simulink model "galipeur"  (R2017a)
settings: Solver=FixedStepAuto  StartTime=0.0  StopTime=inf  FixedStep=0.01  MaxStep=0.05  RelTol=1e-3
model workspace (MAT data in the model file):
  Jz = 3
  alpha0 = 1.57079632679
  alpha1 = 3.66519142919
  alpha2 = 5.75958653158
  mass = 3
  radius = 0.3
undefined symbols (not defined in the file): DiscIntNeverNeededParam
libraries: galipeur_lib x6, simulink x1
settings Model: Creator=jdam  LastModifiedBy=jdam
settings SolverCC: InitialStep=0.05

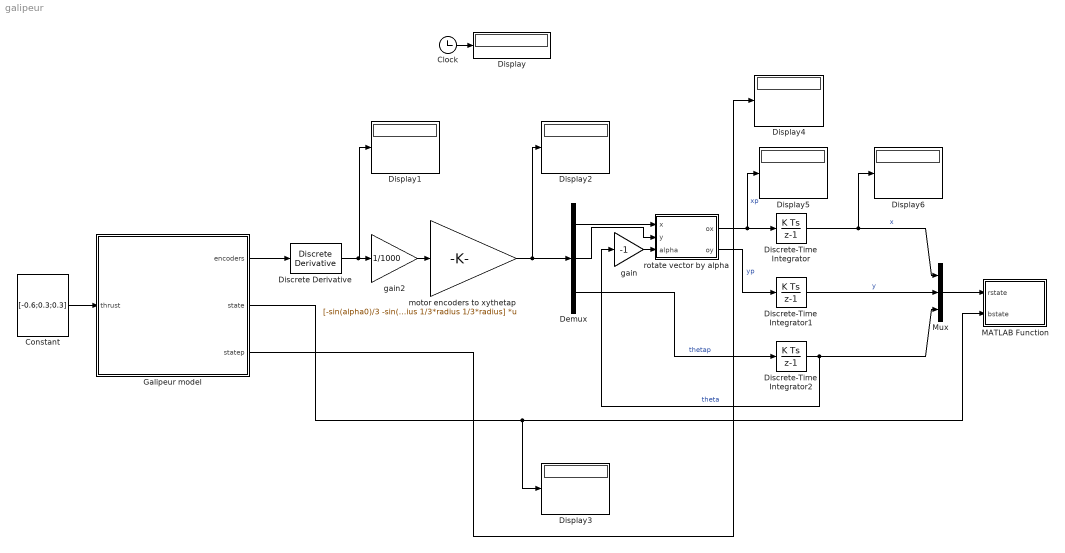
== system galipeur ==
  Clock : Clock
  Constant : Constant  Value=[-0.6;0.3;0.3]  VectorParams1D=off
  Demux : Demux  Outputs=3
  Discrete Derivative : simulink/Discrete/Discrete Derivative  gainval=1.0  ICPrevScaledInput=0.0  OutMin=[]  OutMax=[]  OutDataType=fixdt(1, 16)  OutScaling=2^-10  DoSatur=off
  Discrete-Time Integrator : DiscreteIntegrator  InitialConditionSetting=State (most efficient)  SampleTime=-1  ICPrevOutput=DiscIntNeverNeededParam  ICPrevScaledInput=DiscIntNeverNeededParam
  Discrete-Time Integrator1 : DiscreteIntegrator  InitialConditionSetting=State (most efficient)  SampleTime=-1  ICPrevOutput=DiscIntNeverNeededParam  ICPrevScaledInput=DiscIntNeverNeededParam
  Discrete-Time Integrator2 : DiscreteIntegrator  InitialConditionSetting=State (most efficient)  SampleTime=-1  ICPrevOutput=DiscIntNeverNeededParam  ICPrevScaledInput=DiscIntNeverNeededParam
  Display{,1..6} (7 alike) : Display
  Galipeur model : Subsystem
  MATLAB Function : MATLAB Function  TreatAsAtomicUnit=on
  Mux : Mux  Inputs=3
  gain : Gain  Gain=-1
  gain2 : Gain  Gain=1/1000
  motor encoders to xythetap : Gain  Gain=[-sin(alpha0)/3 -sin(alpha1)/3 -sin(alpha2)/3; cos(alpha0)/3 cos(alpha1)/3 cos(alpha2)/3; 1/3*radius 1/3*radius 1/3*radius]  Multiplication=Matrix(K*u) (u vector)
  rotate vector by alpha : MATLAB Function  TreatAsAtomicUnit=on
  wires:
  Clock/1 -> Display/1
  Constant/1 -> Galipeur model/1(thrust)
  Galipeur model/1(encoders) -> Discrete Derivative/1
  Discrete Derivative/1 -> Display1/1, gain2/1
  Demux/1 -> rotate vector by alpha/1(x)
  Demux/2 -> rotate vector by alpha/2(y)
  rotate vector by alpha/1(ox) -> Display5/1, Discrete-Time Integrator/1  "xp"
  rotate vector by alpha/2(oy) -> Discrete-Time Integrator1/1  "yp"
  gain/1 -> rotate vector by alpha/3(alpha)
  Discrete-Time Integrator/1 -> Display6/1, Mux/1  "x"
  Demux/3 -> Discrete-Time Integrator2/1  "thetap"
  Discrete-Time Integrator1/1 -> Mux/2  "y"
  Discrete-Time Integrator2/1 -> gain/1, Mux/3  "theta"
  motor encoders to xythetap/1 -> Display2/1, Demux/1
  gain2/1 -> motor encoders to xythetap/1
  Mux/1 -> MATLAB Function/1(rstate)
  Galipeur model/2(state) -> Display3/1, MATLAB Function/2(bstate)
  Galipeur model/3(statep) -> Display4/1

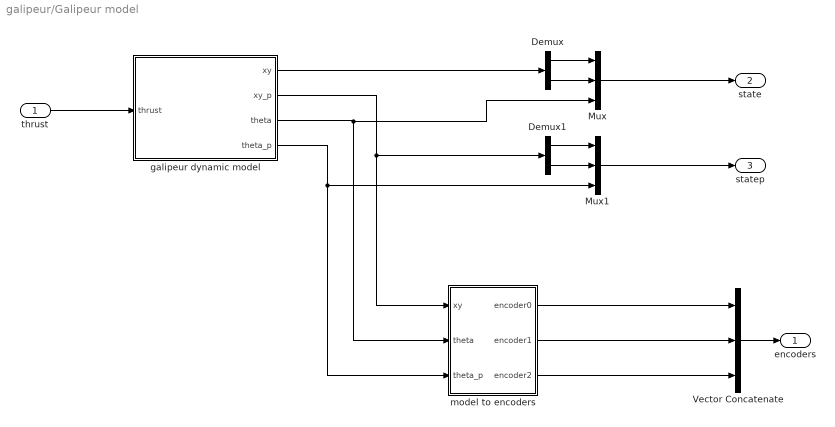
== system galipeur/Galipeur model ==
  thrust : Inport
  Demux : Demux  Outputs=2
  Demux1 : Demux  Outputs=2
  Mux : Mux  Inputs=3
  Mux1 : Mux  Inputs=3
  Vector Concatenate : Concatenate  NumInputs=3
  galipeur dynamic model : Subsystem
  model to encoders : Subsystem
  encoders : Outport
  state : Outport  Port=2
  statep : Outport  Port=3
  wires:
  galipeur dynamic model/3(theta) -> Mux/3, model to encoders/2(theta)
  model to encoders/1(encoder0) -> Vector Concatenate/1
  model to encoders/3(encoder2) -> Vector Concatenate/3
  model to encoders/2(encoder1) -> Vector Concatenate/2
  thrust/1 -> galipeur dynamic model/1(thrust)
  Vector Concatenate/1 -> encoders/1
  Demux/2 -> Mux/2
  Demux/1 -> Mux/1
  galipeur dynamic model/1("xy ") -> Demux/1
  Mux/1 -> state/1
  Demux1/1 -> Mux1/1
  galipeur dynamic model/2(xy_p) -> Demux1/1, model to encoders/1(xy)
  Demux1/2 -> Mux1/2
  galipeur dynamic model/4(theta_p) -> model to encoders/3(theta_p), Mux1/3
  Mux1/1 -> statep/1

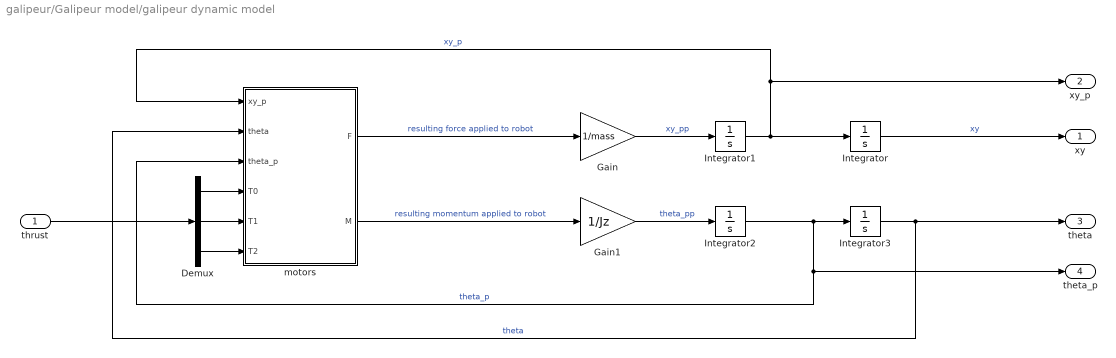
== system galipeur/Galipeur model/galipeur dynamic model ==
  thrust : Inport
  Demux : Demux  Outputs=3
  Gain : Gain  Gain=1/mass
  Gain1 : Gain  Gain=1/Jz
  Integrator{,1..3} (4 alike) : Integrator
  motors : Subsystem
  "xy " : Outport
  xy_p : Outport  Port=2
  theta : Outport  Port=3
  theta_p : Outport  Port=4
  wires:
  Integrator2/1 -> theta_p/1, motors/3(theta_p), Integrator3/1  "theta_p"
  Gain1/1 -> Integrator2/1  "theta_pp"
  Gain/1 -> Integrator1/1  "xy_pp"
  Integrator1/1 -> xy_p/1, motors/1(xy_p), Integrator/1  "xy_p"
  Integrator3/1 -> theta/1, motors/2(theta)  "theta"
  Integrator/1 -> "xy "/1  "xy"
  motors/1(F) -> Gain/1  "resulting force applied to robot"
  motors/2(M) -> Gain1/1  "resulting momentum applied to robot"
  Demux/1 -> motors/4(T0)
  Demux/2 -> motors/5(T1)
  Demux/3 -> motors/6(T2)
  thrust/1 -> Demux/1

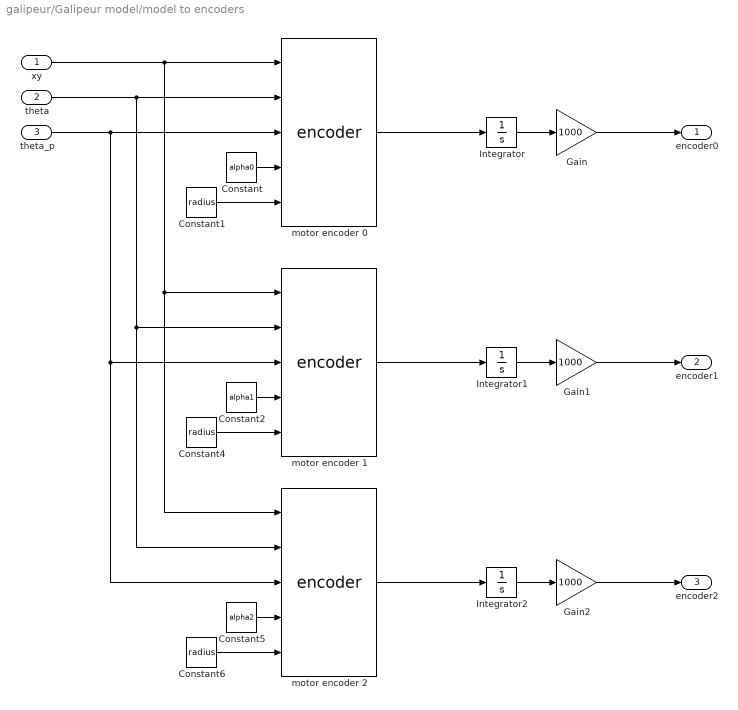
== system galipeur/Galipeur model/model to encoders ==
  xy : Inport
  theta : Inport  Port=2
  theta_p : Inport  Port=3
  Constant : Constant  Value=alpha0
  Constant1 : Constant  Value=radius
  Constant2 : Constant  Value=alpha1
  Constant4 : Constant  Value=radius
  Constant5 : Constant  Value=alpha2
  Constant6 : Constant  Value=radius
  Gain : Gain  Gain=1000
  Gain1 : Gain  Gain=1000
  Gain2 : Gain  Gain=1000
  Integrator : Integrator
  Integrator1 : Integrator
  Integrator2 : Integrator
  motor encoder 0 : galipeur_lib/encoder
  motor encoder 1 : galipeur_lib/encoder
  motor encoder 2 : galipeur_lib/encoder
  encoder0 : Outport
  encoder1 : Outport  Port=2
  encoder2 : Outport  Port=3
  wires:
  Constant2/1 -> motor encoder 1/4
  Gain1/1 -> encoder1/1
  xy/1 -> motor encoder 2/1, motor encoder 1/1, motor encoder 0/1
  Constant1/1 -> motor encoder 0/5
  Constant5/1 -> motor encoder 2/4
  motor encoder 0/1 -> Integrator/1
  Constant6/1 -> motor encoder 2/5
  Constant4/1 -> motor encoder 1/5
  Gain/1 -> encoder0/1
  motor encoder 2/1 -> Integrator2/1
  Constant/1 -> motor encoder 0/4
  Integrator/1 -> Gain/1
  theta/1 -> motor encoder 2/2, motor encoder 1/2, motor encoder 0/2
  Integrator2/1 -> Gain2/1
  Integrator1/1 -> Gain1/1
  theta_p/1 -> motor encoder 0/3, motor encoder 2/3, motor encoder 1/3
  motor encoder 1/1 -> Integrator1/1
  Gain2/1 -> encoder2/1

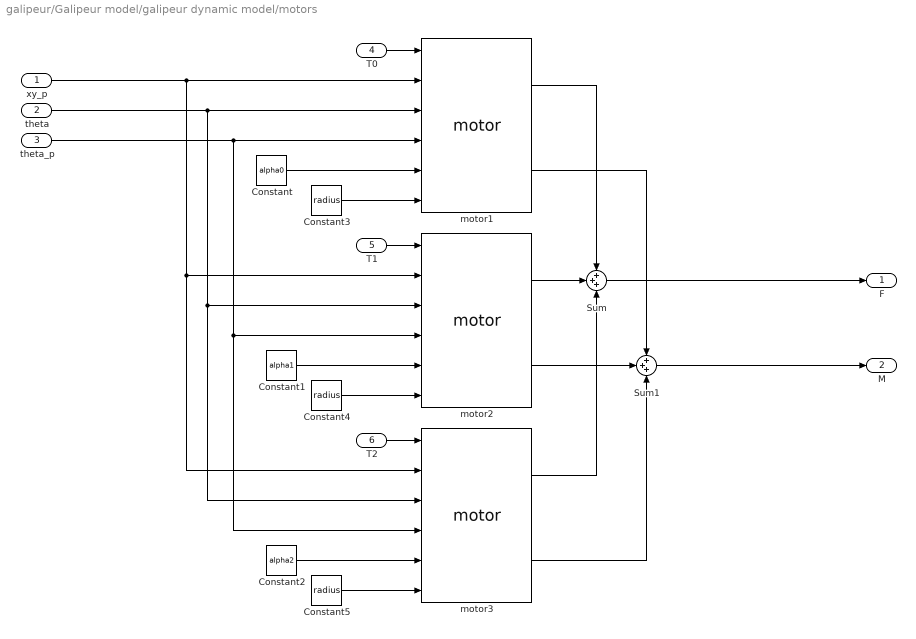
== system galipeur/Galipeur model/galipeur dynamic model/motors ==
  xy_p : Inport
  theta : Inport  Port=2
  theta_p : Inport  Port=3
  T0 : Inport  Port=4
  T1 : Inport  Port=5
  T2 : Inport  Port=6
  Constant : Constant  Value=alpha0
  Constant1 : Constant  Value=alpha1
  Constant2 : Constant  Value=alpha2
  Constant3 : Constant  Value=radius
  Constant4 : Constant  Value=radius
  Constant5 : Constant  Value=radius
  Sum : Sum  Inputs=+++
  Sum1 : Sum  Inputs=+++
  motor1 : galipeur_lib/motor
  motor2 : galipeur_lib/motor
  motor3 : galipeur_lib/motor
  F : Outport
  M : Outport  Port=2
  wires:
  motor1/2 -> Sum1/1
  Constant4/1 -> motor2/6
  xy_p/1 -> motor2/2, motor3/2, motor1/2
  theta_p/1 -> motor1/4, motor3/4, motor2/4
  Constant5/1 -> motor3/6
  Constant2/1 -> motor3/5
  Sum/1 -> F/1
  motor2/1 -> Sum/2
  motor1/1 -> Sum/1
  Constant/1 -> motor1/5
  motor3/1 -> Sum/3
  theta/1 -> motor2/3, motor3/3, motor1/3
  motor3/2 -> Sum1/3
  motor2/2 -> Sum1/2
  Sum1/1 -> M/1
  Constant1/1 -> motor2/5
  Constant3/1 -> motor1/6
  T0/1 -> motor1/1
  T1/1 -> motor2/1
  T2/1 -> motor3/1

== matlab function galipeur/rotate vector by alpha ==
  data: x input; ox output; y input; alpha input; oy output
function [ox,oy]= fcn(x,y,alpha)
% rotate (x,y) vector by alpha

in = [x;y];
R = [cos(alpha) -sin(alpha);
     sin(alpha) cos(alpha)];
out = R*in;
ox = out(1);
oy = out(2);

== matlab function galipeur/MATLAB Function ==
  data: rstate input; bstate input
function fcn(rstate,bstate)
% plot robot
state=rstate;
xy=[state(1);state(2)];
theta=[state(3)];
a0=pi/2;
a1=pi/2 + 2*pi/3;
a2=pi/2 + 4*pi/3;
R=0.3;
p0 = xy + R*[cos(a0+theta); sin(a0+theta)];
p1 = xy + R*[cos(a1+theta); sin(a1+theta)];
p2 = xy + R*[cos(a2+theta); sin(a2+theta)];


hold off
plot([p0(1) p1(1) p2(1) p0(1)],[p0(2) p1(2) p2(2) p0(2)],'r-')
xlim([-3 3])
ylim([-3 3])

state=bstate;
xy=[state(1);state(2)];
theta=[state(3)];
a0=pi/2;
a1=pi/2 + 2*pi/3;
a2=pi/2 + 4*pi/3;
R=0.3;
p0 = xy + R*[cos(a0+theta); sin(a0+theta)];
p1 = xy + R*[cos(a1+theta); sin(a1+theta)];
p2 = xy + R*[cos(a2+theta); sin(a2+theta)];

hold on
plot([p0(1) p1(1) p2(1) p0(1)],[p0(2) p1(2) p2(2) p0(2)],'b-')
xlim([-3 3])
ylim([-3 3])
